simulink model "punto3"  (R2015b)
settings: Solver=VariableStepAuto  StartTime=0.0  StopTime=10.0  RelTol=1e-3
undefined symbols (not defined in the file): punto3
libraries: fuzblock x1
settings Model: Creator=TutyFruty  LastModifiedBy=TutyFruty

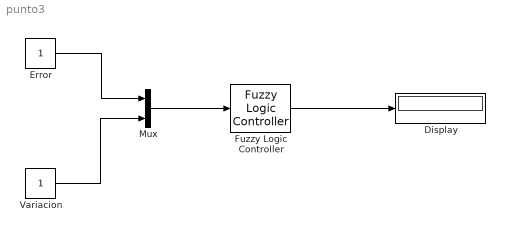
== system punto3 ==
  Display : Display
      settings: Decimation=2
  Error : Constant
  Fuzzy Logic Controller : fuzblock/Fuzzy Logic  Controller  fis=[punto3.fis]
  Mux : Mux  Inputs=2
  Variacion : Constant
  wires:
  Error/1 -> Mux/1
  Variacion/1 -> Mux/2
  Mux/1 -> Fuzzy Logic Controller/1
  Fuzzy Logic Controller/1 -> Display/1
